simulink model "Week2_Problem3"  (R2020b)
settings: Solver=VariableStepAuto  StartTime=0.0  StopTime=10.0  RelTol=1e-3
settings Model: Creator=sai  LastModifiedBy=sai

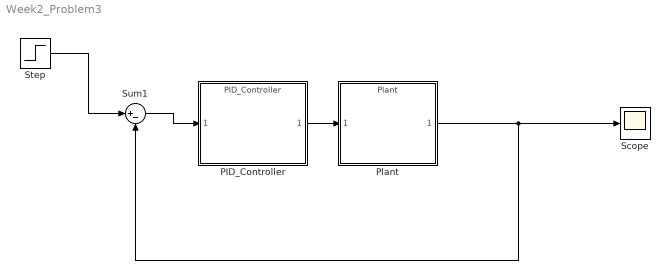
== system Week2_Problem3 ==
  PID_Controller : ModelReference  ModelNameDialog=PID_Controller  ModelReferenceVersion=1.2
  Plant : ModelReference  ModelNameDialog=Plant  ModelReferenceVersion=1.3
  Scope : Scope
  Step : Step  Time=0  After=500  SampleTime=0
  Sum1 : Sum  Inputs=|+-
  wires:
  Plant/1 -> Scope/1, Sum1/2
  Step/1 -> Sum1/1
  PID_Controller/1 -> Plant/1
  Sum1/1 -> PID_Controller/1
